simulink model "Lab6_ciagly_2015a"  (R2015a)
settings: Solver=ode3  SolverMode=SingleTasking  StartTime=0.0  StopTime=10.0  FixedStep=0.01  RelTol=1e-3
libraries: cstblocks x2
settings Model: CovMetricSettings=dwe  CovHtmlReporting=off  covSaveCumulativeToWorkspaceVar=off  CovSaveSingleToWorkspaceVar=off  CovExternalEMLEnable=on  Creator=ishiguro  LastModifiedBy=ishiguro
settings DataIOCC: LimitDataPoints=off  SaveFormat=Dataset
settings DebuggingCC: SFUnexpectedBacktrackingDiag=error  SFNoUnconditionalDefaultTransitionDiag=error
settings HardwareCC: ProdBitPerPointer=64  ProdLargestAtomicFloat=Float  ProdIntDivRoundTo=Zero  ProdEndianess=LittleEndian  ProdHWDeviceType=Specified
settings ModelReferenceCC: PropagateSignalLabelsOutOfModel=on
settings GRTTargetCC: TargetLangStandard=C99 (ISO)  GeneratePreprocessorConditionals=Use local settings

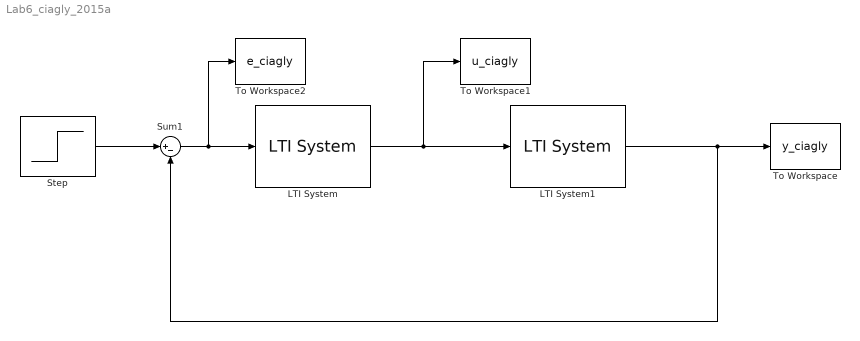
== system Lab6_ciagly_2015a ==
  LTI System : cstblocks/LTI System  sys=Kr  IC=[]
  LTI System1 : cstblocks/LTI System  sys=K  IC=[]
  Step : Step  Time=0  SampleTime=0
  Sum1 : Sum  Inputs=|+-
  To Workspace : ToWorkspace  VariableName=y_ciagly  SampleTime=-1
  To Workspace1 : ToWorkspace  VariableName=u_ciagly  SampleTime=-1
  To Workspace2 : ToWorkspace  VariableName=e_ciagly  SampleTime=-1
  wires:
  Step/1 -> Sum1/1
  LTI System1/1 -> To Workspace/1, Sum1/2
  LTI System/1 -> To Workspace1/1, LTI System1/1
  Sum1/1 -> To Workspace2/1, LTI System/1
